simulink model "mmcontrollerVerification_th"  (R2018b)
settings: Solver=ode15s  StartTime=0.0  StopTime=duration_s  MaxStep=5  RelTol=1e-3  AbsTol=1e-3
undefined symbols (not defined in the file or in its folder): ini_euler_ang, ini_O_Vcm_o, ini_OwB, ini_Rcm_o, sim_param
libraries: thrAttachPtKinematics_ul x3, allActuatorCtrl_cl x1, ayazFlow_cl x1, threeTethers_cl x1, eulAng2RotMat_ul x1, ayazWinches_cl x1, threeTetherGroundStation_cl x1
settings Model: Creator=mcobb  LastModifiedBy=jldanie5

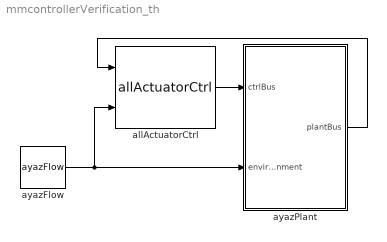
== system mmcontrollerVerification_th ==
  allActuatorCtrl : allActuatorCtrl_cl/allActuatorCtrl  SystemSampleTime=-1
  ayazFlow : ayazFlow_cl/ayazFlow  SystemSampleTime=-1
  ayazPlant : Subsystem
  wires:
  allActuatorCtrl/1 -> ayazPlant/1(ctrlBus)
  ayazPlant/1(plantBus) -> allActuatorCtrl/1
  ayazFlow/1 -> allActuatorCtrl/2, ayazPlant/2(environment)

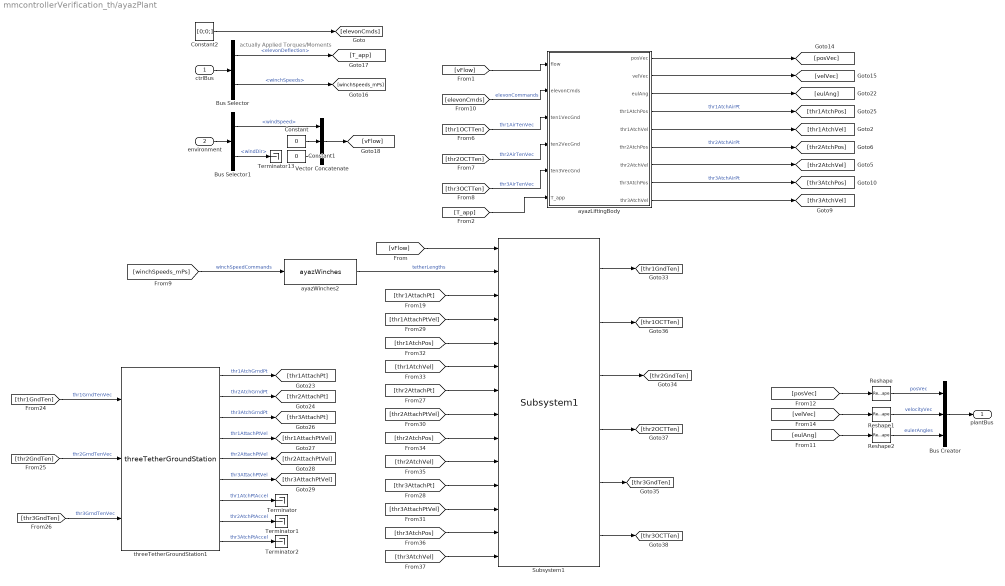
== system mmcontrollerVerification_th/ayazPlant ==
  note: actually Applied Torques/Moments
  ctrlBus : Inport  OutDataTypeStr=Bus: ctrlBus
  environment : Inport  Port=2  OutDataTypeStr=Bus: envBus
  Bus Creator : BusCreator  Inputs=3  OutDataTypeStr=Bus: plantBus
  Bus Selector : BusSelector  OutputSignals=elevonDeflection,winchSpeeds
  Bus Selector1 : BusSelector  OutputSignals=windSpeed,windDir
  Constant : Constant  Value=0
  Constant1 : Constant  Value=0
  Constant2 : Constant  Value=[0;0;]
  Reshape : Reshape  OutputDimensionality=Column vector (2-D)
  Reshape1 : Reshape  OutputDimensionality=Column vector (2-D)
  Reshape2 : Reshape  OutputDimensionality=Column vector (2-D)
  Subsystem1 : threeTethers_cl/Subsystem1  SystemSampleTime=-1
  Terminator{,1..2,13} (4 alike) : Terminator
  Vector Concatenate : Concatenate  NumInputs=3
  ayazLiftingBody : Subsystem
  ayazWinches2 : ayazWinches_cl/ayazWinches  maxSpeed=maxWinchSpeed  maxAccel=maxWinchAccel  timeConst=1  tetherLengths=unstretched_l
  threeTetherGroundStation1 : threeTetherGroundStation_cl/threeTetherGroundStation  fixed=1  J=sim_param.platform_param.platform_Izz  b=sim_param.platform_param.platform_damping  posVec=[0 0 0]  thr1AttachPt=sim_param.tether_imp_nodes.R11_g  thr2AttachPt=sim_param.tether_imp_nodes.R21_g  thr3AttachPt=sim_param.tether_imp_nodes.R31_g  initAngPos=ini_platform_ang  initAngVel=ini_platform_vel
  plantBus : Outport  OutDataTypeStr=Bus: plantBus
  wires:
  [eulAng] -> Reshape2/1
  [velVec] -> Reshape1/1
  [posVec] -> Reshape/1
  Subsystem1/5 -> [thr3GndTen]
  Subsystem1/6 -> [thr3OCTTen]
  Subsystem1/4 -> [thr2OCTTen]
  Subsystem1/3 -> [thr2GndTen]
  Subsystem1/2 -> [thr1OCTTen]
  Subsystem1/1 -> [thr1GndTen]
  [thr1AtchVel] -> Subsystem1/6
  [thr2AtchPos] -> Subsystem1/9
  [thr2AtchVel] -> Subsystem1/10
  [thr3AtchPos] -> Subsystem1/13
  [thr3AtchVel] -> Subsystem1/14
  [thr1AtchPos] -> Subsystem1/5
  [thr1AttachPtVel] -> Subsystem1/4
  [thr2AttachPtVel] -> Subsystem1/8
  [thr3AttachPtVel] -> Subsystem1/12
  [thr3AttachPt] -> Subsystem1/11
  [thr2AttachPt] -> Subsystem1/7
  [thr1AttachPt] -> Subsystem1/3
  [vFlow] -> Subsystem1/1
  threeTetherGroundStation1/7 -> Terminator/1  "thr1AtchPtAccel"
  [thr1GndTen] -> threeTetherGroundStation1/1  "thr1GrndTenVec"
  [thr3GndTen] -> threeTetherGroundStation1/3  "thr3GrndTenVec"
  [winchSpeeds_mPs] -> ayazWinches2/1  "winchSpeedCommands"
  [thr2GndTen] -> threeTetherGroundStation1/2  "thr2GrndTenVec"
  ayazWinches2/1 -> Subsystem1/2  "tetherLengths"
  threeTetherGroundStation1/1 -> [thr1AttachPt]  "thr1AtchGrndPt"
  threeTetherGroundStation1/3 -> [thr3AttachPt]  "thr3AtchGrndPt"
  threeTetherGroundStation1/2 -> [thr2AttachPt]  "thr2AtchGrndPt"
  threeTetherGroundStation1/4 -> [thr1AttachPtVel]  "thr1AttachPtVel"
  threeTetherGroundStation1/8 -> Terminator1/1  "thr2AtchPtAccel"
  threeTetherGroundStation1/5 -> [thr2AttachPtVel]  "thr2AttachPtVel"
  threeTetherGroundStation1/6 -> [thr3AttachPtVel]  "thr3AttachPtVel"
  threeTetherGroundStation1/9 -> Terminator2/1  "thr3AtchPtAccel"
  ayazLiftingBody/9(thr3AtchVel) -> [thr3AtchVel]
  ayazLiftingBody/8(thr3AtchPos) -> [thr3AtchPos]  "thr3AtchAirPt"
  ayazLiftingBody/7(thr2AtchVel) -> [thr2AtchVel]
  ayazLiftingBody/6(thr2AtchPos) -> [thr2AtchPos]  "thr2AtchAirPt"
  ayazLiftingBody/5(thr1AtchVel) -> [thr1AtchVel]
  ayazLiftingBody/4(thr1AtchPos) -> [thr1AtchPos]  "thr1AtchAirPt"
  ayazLiftingBody/3(eulAng) -> [eulAng]
  Constant1/1 -> Vector Concatenate/3
  Constant/1 -> Vector Concatenate/2
  Vector Concatenate/1 -> [vFlow]
  Reshape1/1 -> Bus Creator/2  "velocityVec"
  Reshape2/1 -> Bus Creator/3  "eulerAngles"
  Reshape/1 -> Bus Creator/1  "posVec"
  Bus Creator/1 -> plantBus/1
  Bus Selector/2 -> [winchSpeeds_mPs]  "<winchSpeeds>"
  Bus Selector1/1 -> Vector Concatenate/1  "<windSpeed>"
  Bus Selector/1 -> [T_app]  "<elevonDeflection>"
  Bus Selector1/2 -> Terminator13/1  "<windDir>"
  ctrlBus/1 -> Bus Selector/1
  environment/1 -> Bus Selector1/1
  [elevonCmds] -> ayazLiftingBody/2(elevonCmds)  "elevonCommands"
  [thr3OCTTen] -> ayazLiftingBody/5(ten3VecGnd)  "thr3AirTenVec"
  [thr2OCTTen] -> ayazLiftingBody/4(ten2VecGnd)  "thr2AirTenVec"
  [thr1OCTTen] -> ayazLiftingBody/3(ten1VecGnd)  "thr1AirTenVec"
  [vFlow] -> ayazLiftingBody/1(flow)
  ayazLiftingBody/2(velVec) -> [velVec]
  ayazLiftingBody/1("posVec ") -> [posVec]
  [T_app] -> ayazLiftingBody/6(T_app)
  Constant2/1 -> [elevonCmds]

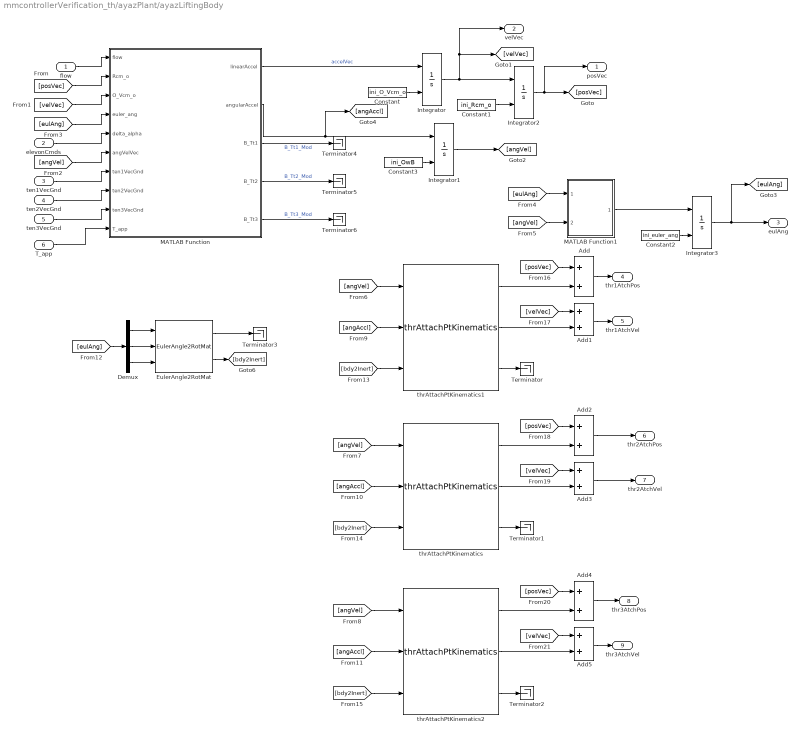
== system mmcontrollerVerification_th/ayazPlant/ayazLiftingBody ==
  flow : Inport
  elevonCmds : Inport  Port=2
  ten1VecGnd : Inport  Port=3
  ten2VecGnd : Inport  Port=4
  ten3VecGnd : Inport  Port=5
  T_app : Inport  Port=6
  Add{,1..5} (6 alike) : Sum
  Constant : Constant  Value=ini_O_Vcm_o
  Constant1 : Constant  Value=ini_Rcm_o
  Constant2 : Constant  Value=ini_euler_ang
  Constant3 : Constant  Value=ini_OwB
  Demux : Demux  Outputs=3
  EulerAngle2RotMat : eulAng2RotMat_ul/EulerAngle2RotMat  SystemSampleTime=-1
  Integrator{,1..3} (4 alike) : Integrator  InitialConditionSource=external
  MATLAB Function : MATLAB Function  TreatAsAtomicUnit=on
  MATLAB Function1 : MATLAB Function  TreatAsAtomicUnit=on
  Terminator{,1..6} (7 alike) : Terminator
  thrAttachPtKinematics : thrAttachPtKinematics_ul/thrAttachPtKinematics  theAtchPosVec=sim_param.tether_imp_nodes.R2n_cm
  thrAttachPtKinematics1 : thrAttachPtKinematics_ul/thrAttachPtKinematics  theAtchPosVec=sim_param.tether_imp_nodes.R1n_cm
  thrAttachPtKinematics2 : thrAttachPtKinematics_ul/thrAttachPtKinematics  theAtchPosVec=sim_param.tether_imp_nodes.R3n_cm
  "posVec " : Outport
  velVec : Outport  Port=2
  eulAng : Outport  Port=3
  thr1AtchPos : Outport  Port=4
  thr1AtchVel : Outport  Port=5
  thr2AtchPos : Outport  Port=6
  thr2AtchVel : Outport  Port=7
  thr3AtchPos : Outport  Port=8
  thr3AtchVel : Outport  Port=9
  wires:
  MATLAB Function/5(B_Tt3) -> Terminator6/1  "B_Tt3_Mod"
  MATLAB Function/4(B_Tt2) -> Terminator5/1  "B_Tt2_Mod"
  MATLAB Function/3(B_Tt1) -> Terminator4/1  "B_Tt1_Mod"
  Add4/1 -> thr3AtchPos/1
  Add5/1 -> thr3AtchVel/1
  [velVec] -> Add5/1
  [posVec] -> Add4/1
  thrAttachPtKinematics2/2 -> Add5/2
  thrAttachPtKinematics2/1 -> Add4/2
  Add3/1 -> thr2AtchVel/1
  Add2/1 -> thr2AtchPos/1
  thrAttachPtKinematics/1 -> Add2/2
  thrAttachPtKinematics/2 -> Add3/2
  [posVec] -> Add2/1
  [velVec] -> Add3/1
  Add1/1 -> thr1AtchVel/1
  [velVec] -> Add1/1
  [posVec] -> Add/1
  Add/1 -> thr1AtchPos/1
  EulerAngle2RotMat/1 -> Terminator3/1
  thrAttachPtKinematics2/3 -> Terminator2/1
  thrAttachPtKinematics/3 -> Terminator1/1
  thrAttachPtKinematics1/3 -> Terminator/1
  thrAttachPtKinematics1/2 -> Add1/2
  thrAttachPtKinematics1/1 -> Add/2
  [bdy2Inert] -> thrAttachPtKinematics2/3
  [bdy2Inert] -> thrAttachPtKinematics/3
  [bdy2Inert] -> thrAttachPtKinematics1/3
  EulerAngle2RotMat/2 -> [bdy2Inert]
  Demux/3 -> EulerAngle2RotMat/3
  Demux/1 -> EulerAngle2RotMat/1
  Demux/2 -> EulerAngle2RotMat/2
  [eulAng] -> Demux/1
  [angAccl] -> thrAttachPtKinematics2/2
  [angAccl] -> thrAttachPtKinematics/2
  [angAccl] -> thrAttachPtKinematics1/2
  [angVel] -> thrAttachPtKinematics2/1
  [angVel] -> thrAttachPtKinematics/1
  [angVel] -> thrAttachPtKinematics1/1
  MATLAB Function1/1(eulAngDeriv) -> Integrator3/1
  [angVel] -> MATLAB Function1/2(angVel)
  [eulAng] -> MATLAB Function1/1(eulAng)
  Constant3/1 -> Integrator1/2
  Constant2/1 -> Integrator3/2
  Constant1/1 -> Integrator2/2
  Constant/1 -> Integrator/2
  elevonCmds/1 -> MATLAB Function/5(delta_alpha)
  flow/1 -> MATLAB Function/1(flow)
  MATLAB Function/1(linearAccel) -> Integrator/1  "accelVec"
  MATLAB Function/2(angularAccel) -> Integrator1/1, [angAccl]
  Integrator1/1 -> [angVel]
  Integrator/1 -> Integrator2/1, [velVec], velVec/1
  Integrator2/1 -> [posVec], "posVec "/1
  [posVec] -> MATLAB Function/2(Rcm_o)
  [velVec] -> MATLAB Function/3(O_Vcm_o)
  Integrator3/1 -> [eulAng], eulAng/1
  [angVel] -> MATLAB Function/6(angVelVec)
  [eulAng] -> MATLAB Function/4(euler_ang)
  ten1VecGnd/1 -> MATLAB Function/7(ten1VecGnd)
  ten2VecGnd/1 -> MATLAB Function/8(ten2VecGnd)
  ten3VecGnd/1 -> MATLAB Function/9(ten3VecGnd)
  T_app/1 -> MATLAB Function/10(T_app)

== matlab function mmcontrollerVerification_th/ayazPlant/ayazLiftingBody/MATLAB Function ==
  data: sim_param parameter; flow input; linearAccel output size=[3 1]; Rcm_o input; O_Vcm_o input; euler_ang input; delta_alpha input; angVelVec input; angularAccel output size=[3 1]; ten1VecGnd input; ten2VecGnd input; ten3VecGnd input; B_Tt1 output; B_Tt2 output; B_Tt3 output; T_app input
function [linearAccel, angularAccel,B_Tt1,B_Tt2,B_Tt3] = B_F_and_T_aero(sim_param,flow,Rcm_o,...
    O_Vcm_o,euler_ang,delta_alpha,angVelVec,ten1VecGnd,ten2VecGnd,...
    ten3VecGnd,T_app)
%% extracting values from sim parameters structure
N = sim_param.N;

env_param = sim_param.env_param;
geom_param = sim_param.geom_param;
aero_param = sim_param.aero_param;
turbine_param = sim_param.turbine_param;
tether_param = sim_param.tether_param;
tether_imp_nodes = sim_param.tether_imp_nodes;


m = geom_param.mass;
m_added = geom_param.m_added;
g = env_param.grav;
% rho = env_param.density;

% CD_cylinder = tether_param.CD_cylinder;
% tether_youngs = tether_param.tether_youngs;


Rcb_cm = geom_param.center_of_buoy;
% Rac_cm = geom_param.aero_center;
% R1turb_cm = turbine_param.R1turb_cm;
% R2turb_cm = turbine_param.R2turb_cm;


% Rvs_cm = aero_param.Rvs_cm;

R1n_cm = tether_imp_nodes.R1n_cm;
R2n_cm = tether_imp_nodes.R2n_cm;
R3n_cm = tether_imp_nodes.R3n_cm;

% R11_g = tether_imp_nodes.R11_g;
% R21_g = tether_imp_nodes.R21_g;
% R31_g = tether_imp_nodes.R31_g;


% calculate tether masses and spring stiffness
% tether_density = tether_param.tether_density;
% tether_dia = tether_param.tether_diameter;
% zeta = tether_param.damping_ratio;

% tether_masses = ((tether_density*(pi/4)).*tether_dia.^2).*unstretched_l;

%% force calculations
% buoyancy force in the ko direction
fz_buoy = geom_param.F_buoy;

% buoyancy force in the O frame
O_F_buoy = [0;0;fz_buoy];

% gravity force in the ko direction
fz_grav = -m*g;

% gravity force in the O frame
O_F_grav = [0;0;fz_grav];

% calculate aerodynamic forces on the lifting body
aero_F = B_F_and_T_aero(sim_param,flow,Rcm_o,O_Vcm_o,euler_ang,delta_alpha);

B_F_aero_mw = aero_F.B_F_aero_mw;
B_F_aero_VS = aero_F.B_F_aero_VS;
B_F_turb1 = aero_F.B_F_turb1;
B_F_turb2 = aero_F.B_F_turb2;

B_T_aero_mw = aero_F.B_T_aero_mw;
B_T_aero_VS = aero_F.B_T_aero_VS;
B_T_aero_turb = aero_F.B_T_aero_turb;


O_F_aero_mw = oCb*B_F_aero_mw;
O_F_aero_VS = oCb*B_F_aero_VS;
O_F_turb1 = oCb*B_F_turb1;
O_F_turb2 = oCb*B_F_turb2;

% %% forces acting on the center of mass
O_F_ext = O_F_buoy + O_F_grav + O_F_aero_mw + O_F_aero_VS + O_F_turb1 + O_F_turb2 +...
    ten1VecGnd + ten2VecGnd + ten3VecGnd;

mass_matrix = [1/(m+m_added(1)) 0 0;0 1/(m+m_added(2)) 0;0 0 1/(m+m_added(3))];


linearAccel = oCb*(mass_matrix*bCo*O_F_ext);
B_T_buoy = cross(Rcb_cm,(bCo*O_F_buoy));
% torque due to gravity about CM
B_T_grav = [0;0;0];

% torque due to the three tethers in the B frame
B_Tt1 = cross(R1n_cm,(bCo*ten1VecGnd));
B_Tt2 = cross(R2n_cm,(bCo*ten2VecGnd));
B_Tt3 = cross(R3n_cm,(bCo*ten3VecGnd));

B_T_ext = B_T_buoy + B_T_grav + B_T_aero_mw + B_T_aero_VS + B_T_aero_turb + ...
    B_Tt1 + B_Tt2 + B_Tt3;

Tx = B_T_ext(1)+T_app(1);
Ty = B_T_ext(2)+T_app(2);
Tz = B_T_ext(3)+T_app(3);

wx = angVelVec(1);
wy = angVelVec(2);
wz = angVelVec(3);

MI = sim_param.geom_param.MI;
Ixx = MI(1,1);
Iyy = MI(2,2);
Izz = MI(3,3);
Izz_added = sim_param.geom_param.Izz_added;

angularAccel = [...
    (1/Ixx)*(Tx + (Iyy - Izz)*wy*wz);...
    (1/Iyy)*(Ty + (Izz - Ixx)*wx*wz);...
    (1/(Izz+Izz_added))*(Tz + (Ixx - Iyy)*wx*wy)];

end

== matlab function mmcontrollerVerification_th/ayazPlant/ayazLiftingBody/MATLAB Function1 ==
  data: eulAng input; eulAngDeriv output; angVel input
function eulAngDeriv = fcn(eulAng,angVel)

wx = angVel(1);
wy = angVel(2);
wz = angVel(3);

ph = eulAng(1);
th = eulAng(2);

eulAngDeriv = zeros(3,1);
eulAngDeriv(1) = wx + sin(ph)*tan(th)*wy + cos(ph)*tan(th)*wz;
eulAngDeriv(2) = cos(ph)*wy - sin(ph)*wz;
eulAngDeriv(3) = sec(th)*sin(ph)*wy + cos(ph)*sec(th)*wz;
